simulink model "test_lsq_sim4_ok"  (R2020b)
settings: Solver=VariableStepAuto  StartTime=0.0  StopTime=10000  RelTol=1e-3
settings Model: Creator=Mehdi  LastModifiedBy=Mehdi

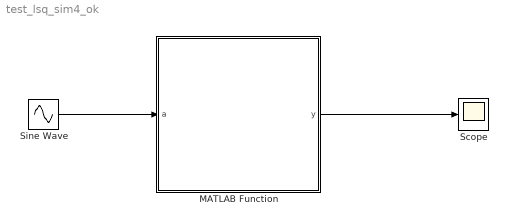
== system test_lsq_sim4_ok ==
  MATLAB Function : MATLAB Function  TreatAsAtomicUnit=on
  Scope : Scope
  Sine Wave : Sin  Amplitude=10  Frequency=0.1  SampleTime=0
  wires:
  MATLAB Function/1(y) -> Scope/1
  Sine Wave/1 -> MATLAB Function/1(a)

== matlab function test_lsq_sim4_ok/MATLAB Function ==
  data: y output; a input
function y=fcn(a)


fun=@(x)sin(x.*x);

x0=[a 2 3];

LB=[0 0 0];
UB=[1000 1000 1000];

options = optimoptions('lsqnonlin','Algorithm','levenberg-marquardt');

y = lsqnonlin(fun,x0,LB,UB,options)';

end
